simulink model "tst_bus_no_signal_names"  (Simulink 8.0)
settings: Solver=ode45  StartTime=0.0  StopTime=10.0  RelTol=1e-3
settings Model: Creator=Marci  LastModifiedBy=Marci

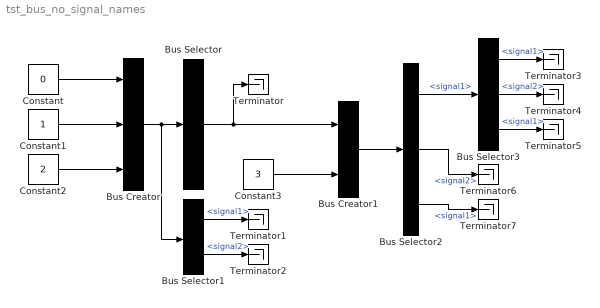
== system tst_bus_no_signal_names ==
  Bus Creator : BusCreator  Inputs=3
  Bus Creator1 : BusCreator  Inputs=2
  Bus Selector : BusSelector  OutputSignals=signal1,signal2  OutputAsBus=on
  Bus Selector1 : BusSelector  OutputSignals=signal1,signal2
  Bus Selector2 : BusSelector  OutputSignals=signal1,signal2,signal1.signal1
  Bus Selector3 : BusSelector  OutputSignals=signal1,signal2,signal1
  Constant : Constant  Value=0
  Constant1 : Constant
  Constant2 : Constant  Value=2
  Constant3 : Constant  Value=3
  Terminator{,1..7} (8 alike) : Terminator
  wires:
  Bus Creator/1 -> Bus Selector1/1, Bus Selector/1
  Constant/1 -> Bus Creator/1
  Constant1/1 -> Bus Creator/2
  Bus Selector1/1 -> Terminator1/1  "<signal1>"
  Bus Selector1/2 -> Terminator2/1  "<signal2>"
  Bus Selector/1 -> Terminator/1, Bus Creator1/1
  Constant3/1 -> Bus Creator1/2
  Bus Creator1/1 -> Bus Selector2/1
  Bus Selector2/1 -> Bus Selector3/1  "<signal1>"
  Bus Selector2/2 -> Terminator6/1  "<signal2>"
  Bus Selector2/3 -> Terminator7/1  "<signal1>"
  Constant2/1 -> Bus Creator/3
  Bus Selector3/1 -> Terminator3/1  "<signal1>"
  Bus Selector3/2 -> Terminator4/1  "<signal2>"
  Bus Selector3/3 -> Terminator5/1  "<signal1>"
